simulink model "validate_controller"  (R2015a)
settings: Solver=FixedStepDiscrete  StartTime=0.0  StopTime=T  FixedStep=0.02  RelTol=1e-3
values from neighbouring files (symbols this model uses):
  A = stateModelMatrices(1:l-1, 1:l-1)    [controller_design_1.m]    (also in controller_design_2.m)
  B = stateModelMatrices(1:l-1, l)    [controller_design_1.m]    (also in controller_design_2.m)
  C = stateModelMatrices(l, 1:l-1)    [controller_design_1.m]    (also in controller_design_2.m)
  D = stateModelMatrices(l, l)    [controller_design_1.m]    (also in controller_design_2.m)
undefined symbols (not defined in the file or in its folder): K
settings Model: Creator=alunos  LastModifiedBy=luisr
settings DataIOCC: LimitDataPoints=off

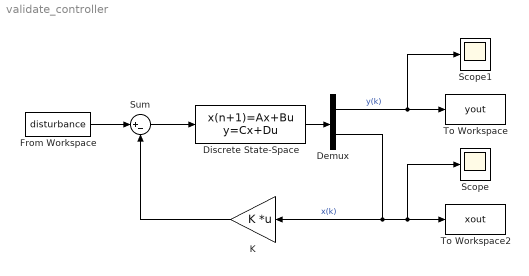
== system validate_controller ==
  Demux : Demux  Outputs=[1 4]
  Discrete State-Space : DiscreteStateSpace  A=A  B=B  C=[C; eye(length(A))]  D=[D; zeros(size(A,1),1)]  SampleTime=0.02
  From Workspace : FromWorkspace  VariableName=disturbance  SampleTime=[0.02,0]
  K : Gain  Gain=K  Multiplication=Matrix(K*u)
  Scope : Scope
      settings: TimeRange=auto  MaxDataPoints=5000  SaveToWorkspace=off  SaveName=ScopeData  YMin=-24.12932  YMax=216.5706  SampleTime=-1
  Scope1 : Scope
      settings: TimeRange=auto  MaxDataPoints=5000  SaveToWorkspace=off  YMin=-24.12932  YMax=216.5706  SampleTime=-1
  Sum : Sum  Inputs=|+-
  To Workspace : ToWorkspace  VariableName=yout  SaveFormat=Structure With Time  SampleTime=-1
  To Workspace2 : ToWorkspace  VariableName=xout  SaveFormat=Structure With Time  SampleTime=-1
  wires:
  From Workspace/1 -> Sum/1
  Sum/1 -> Discrete State-Space/1
  K/1 -> Sum/2
  Demux/2 -> Scope/1, To Workspace2/1, K/1  "x(k)"
  Discrete State-Space/1 -> Demux/1
  Demux/1 -> Scope1/1, To Workspace/1  "y(k)"
